simulink model "Differential_steer_kinematic"  (R2020b)
settings: Solver=FixedStepAuto  StartTime=0.0  StopTime=1000  FixedStep=.0001  MinStep=1E-5  RelTol=1e-3
values from neighbouring files (symbols this model uses):
  delay = 0.15    [Jackal_kinematic_model.m]
undefined symbols (not defined in the file or in its folder): path
libraries: fuzblock x2, robotalgslib x1, simulink x1
settings Model: Creator=12248  LastModifiedBy=mcichon2
settings SFSimCC: CustomCodeUndefinedFunction=UseInterfaceOnly

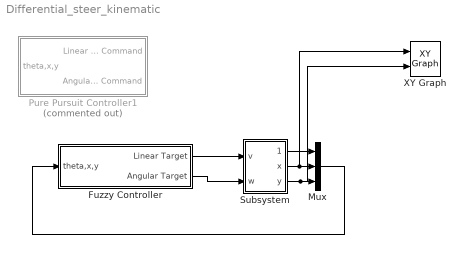
== system Differential_steer_kinematic ==
  Fuzzy Controller : Subsystem
  Mux : Mux  Inputs=3
  Pure Pursuit Controller1 : Subsystem  Commented=on
  Subsystem : Subsystem
  XY Graph : simulink/Sinks/XY Graph  xmin=-10  xmax=10  ymin=-10  ymax=10  st=-1
  wires:
  Mux/1 -> Fuzzy Controller/1(theta,x,y)
  Subsystem/1(theta) -> Mux/1
  Subsystem/2(x) -> XY Graph/1, Mux/2
  Subsystem/3(y) -> XY Graph/2, Mux/3
  Fuzzy Controller/1(Linear Target) -> Subsystem/1(v)
  Fuzzy Controller/2(" Angular Target") -> Subsystem/2(w)

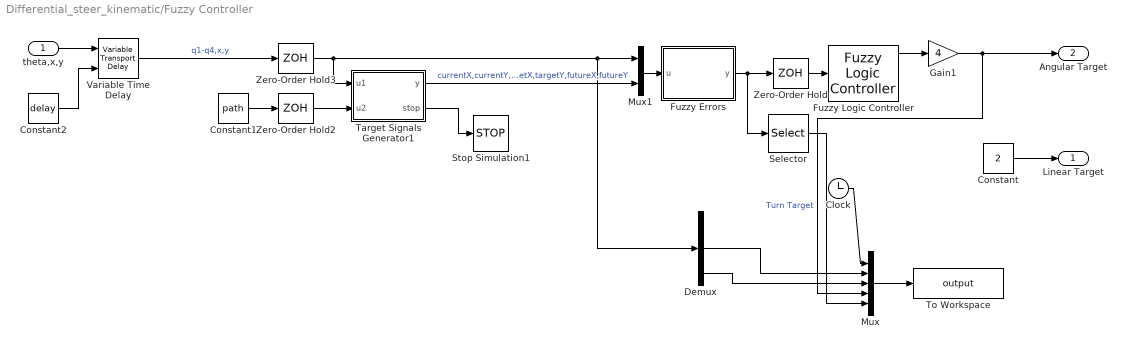
== system Differential_steer_kinematic/Fuzzy Controller ==
  theta,x,y : Inport
  Clock : Clock
  Constant : Constant  Value=2
  Constant1 : Constant  Value=path
  Constant2 : Constant  Value=delay
  Demux : Demux  Outputs=3
  Fuzzy Errors : MATLAB Function  TreatAsAtomicUnit=on
  Fuzzy Logic Controller : fuzblock/Fuzzy Logic  Controller  FIS='fuzzyControlDistNew.fis'  OutputSampleNumber=3000  DataType=double  FuzzifiedInputs=off  RuleFiringStrengths=on  RuleOutputs=off  AggregatedOutputs=on  SimulateUsing=Code generation  OutOfRangeInputValueMessage=warning  NoRuleFiredMessage=warning  EmptyOutputFuzzySetMessage=warning
  Gain1 : Gain  Gain=4
  Mux : Mux  Inputs=5
  Mux1 : Mux  Inputs=2
  Selector : Selector  InputPortWidth=5  IndexOptions=Index vector (dialog)  Indices=[1]  OutputSizes=1
  Stop Simulation1 : Stop
  Target Signals Generator1 : MATLAB Function  TreatAsAtomicUnit=on
  To Workspace : ToWorkspace  VariableName=output  SampleTime=-1
  Variable Time Delay : VariableTransportDelay  MaximumDelay=10
  Zero-Order Hold : ZeroOrderHold  SampleTime=.001
  Zero-Order Hold2 : ZeroOrderHold  SampleTime=.001
  Zero-Order Hold3 : ZeroOrderHold  SampleTime=.001
  Linear Target : Outport  VectorParamsAs1DForOutWhenUnconnected=off
  " Angular Target" : Outport  Port=2  VectorParamsAs1DForOutWhenUnconnected=off
  wires:
  Mux1/1 -> Fuzzy Errors/1(u)
  Variable Time Delay/1 -> Zero-Order Hold3/1  "q1-q4,x,y"
  Target Signals Generator1/1(y) -> Mux1/2  "currentX,currentY,targetX,targetY,futureX,futureY"
  Constant1/1 -> Zero-Order Hold2/1
  Zero-Order Hold2/1 -> Target Signals Generator1/2(u2)
  Target Signals Generator1/2(stop) -> Stop Simulation1/1
  Fuzzy Errors/1(y) -> Selector/1, Zero-Order Hold/1
  Zero-Order Hold/1 -> Fuzzy Logic Controller/1
  Fuzzy Logic Controller/1 -> Gain1/1
  Gain1/1 -> Mux/4, " Angular Target"/1  "Turn Target"
  theta,x,y/1 -> Variable Time Delay/1
  Constant/1 -> Linear Target/1
  Selector/1 -> Mux/5
  Mux/1 -> To Workspace/1
  Zero-Order Hold3/1 -> Target Signals Generator1/1(u1), Demux/1, Mux1/1
  Constant2/1 -> Variable Time Delay/2
  Clock/1 -> Mux/1
  Demux/2 -> Mux/2
  Demux/3 -> Mux/3

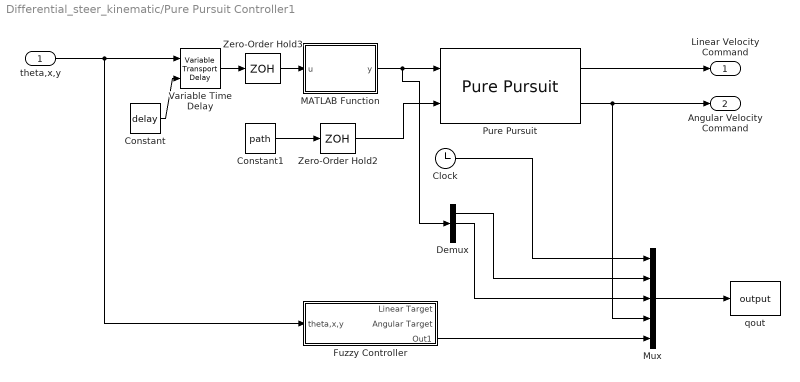
== system Differential_steer_kinematic/Pure Pursuit Controller1 ==
  theta,x,y : Inport
  Clock : Clock
  Constant : Constant  Value=delay
  Constant1 : Constant  Value=path
  Demux : Demux  Outputs=3
  Fuzzy Controller : Subsystem
  MATLAB Function : MATLAB Function  TreatAsAtomicUnit=on
  Mux : Mux  Inputs=5
  Pure Pursuit : robotalgslib/Pure Pursuit  DesiredLinearVelocity=speed  MaxAngularVelocity=4.0  LookaheadDistance=la_dist  TargetDirPort=off  SimulateUsing=Code generation
  Variable Time Delay : VariableTransportDelay  MaximumDelay=10
  Zero-Order Hold2 : ZeroOrderHold  SampleTime=.001
  Zero-Order Hold3 : ZeroOrderHold  SampleTime=.001
  qout : ToWorkspace  VariableName=output  SampleTime=-1
  Linear Velocity Command : Outport  VectorParamsAs1DForOutWhenUnconnected=off
  Angular Velocity Command : Outport  Port=2  VectorParamsAs1DForOutWhenUnconnected=off
  wires:
  Zero-Order Hold3/1 -> MATLAB Function/1(u)
  Constant1/1 -> Zero-Order Hold2/1
  MATLAB Function/1(y) -> Demux/1, Pure Pursuit/1
  Zero-Order Hold2/1 -> Pure Pursuit/2
  Pure Pursuit/2 -> Angular Velocity Command/1, Mux/4
  Variable Time Delay/1 -> Zero-Order Hold3/1
  Pure Pursuit/1 -> Linear Velocity Command/1
  Constant/1 -> Variable Time Delay/2
  Mux/1 -> qout/1
  Clock/1 -> Mux/1
  Fuzzy Controller/3(Out1) -> Mux/5
  theta,x,y/1 -> Fuzzy Controller/1(theta,x,y), Variable Time Delay/1
  Demux/1 -> Mux/2
  Demux/2 -> Mux/3

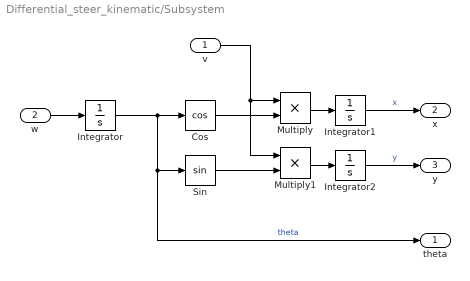
== system Differential_steer_kinematic/Subsystem ==
  v : Inport
  w : Inport  Port=2
  Cos : Trigonometry  Operator=cos
  Integrator : Integrator
  Integrator1 : Integrator
  Integrator2 : Integrator
  Multiply : Product
  Multiply1 : Product
  Sin : Trigonometry
  theta : Outport  VectorParamsAs1DForOutWhenUnconnected=off
  x : Outport  Port=2  VectorParamsAs1DForOutWhenUnconnected=off
  y : Outport  Port=3  VectorParamsAs1DForOutWhenUnconnected=off
  wires:
  Sin/1 -> Multiply1/2
  Multiply1/1 -> Integrator2/1
  Integrator/1 -> theta/1, Sin/1, Cos/1  "theta"
  Cos/1 -> Multiply/2
  Multiply/1 -> Integrator1/1
  Integrator1/1 -> x/1  "x"
  Integrator2/1 -> y/1  "y"
  v/1 -> Multiply1/1, Multiply/1
  w/1 -> Integrator/1

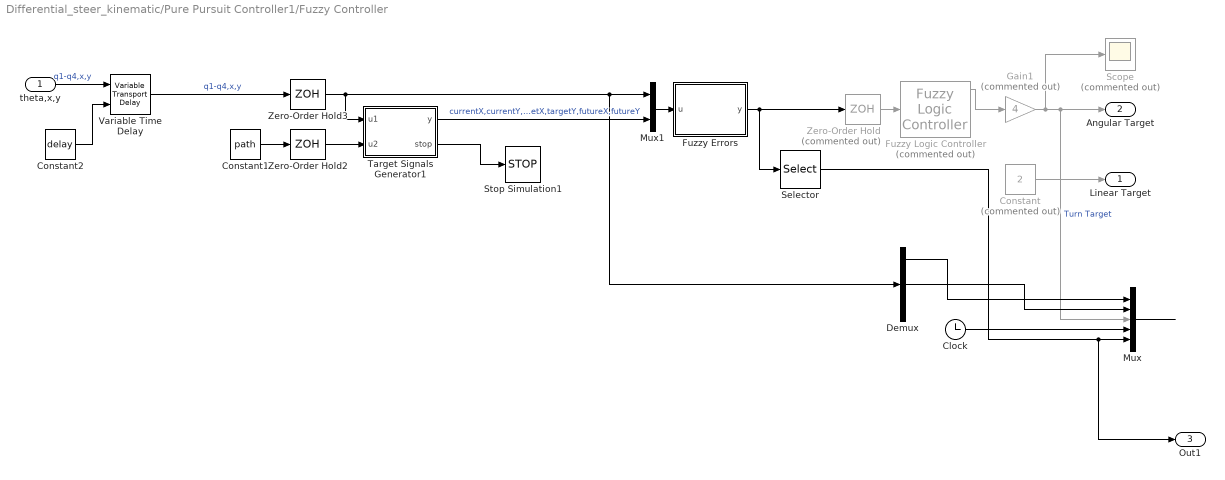
== system Differential_steer_kinematic/Pure Pursuit Controller1/Fuzzy Controller ==
  theta,x,y : Inport
  Clock : Clock
  Constant : Constant  Commented=on  Value=2
  Constant1 : Constant  Value=path
  Constant2 : Constant  Value=delay
  Demux : Demux  Outputs=3
  Fuzzy Errors : MATLAB Function  TreatAsAtomicUnit=on
  Fuzzy Logic Controller : fuzblock/Fuzzy Logic  Controller  Commented=on  FIS='fuzzyControlDistNew.fis'  OutputSampleNumber=3000  DataType=double  FuzzifiedInputs=off  RuleFiringStrengths=on  RuleOutputs=off  AggregatedOutputs=on  SimulateUsing=Code generation  OutOfRangeInputValueMessage=warning  NoRuleFiredMessage=warning  EmptyOutputFuzzySetMessage=warning
  Gain1 : Gain  Commented=on  Gain=4
  Mux : Mux  Inputs=5
  Mux1 : Mux  Inputs=2
  Scope : Scope  Commented=on
  Selector : Selector  InputPortWidth=5  IndexOptions=Index vector (dialog)  Indices=[1]  OutputSizes=1
  Stop Simulation1 : Stop
  Target Signals Generator1 : MATLAB Function  TreatAsAtomicUnit=on
  Variable Time Delay : VariableTransportDelay  MaximumDelay=10
  Zero-Order Hold : ZeroOrderHold  Commented=on  SampleTime=.001
  Zero-Order Hold2 : ZeroOrderHold  SampleTime=.001
  Zero-Order Hold3 : ZeroOrderHold  SampleTime=.001
  Linear Target : Outport  VectorParamsAs1DForOutWhenUnconnected=off
  " Angular Target" : Outport  Port=2  VectorParamsAs1DForOutWhenUnconnected=off
  Out1 : Outport  Port=3
  wires:
  Mux1/1 -> Fuzzy Errors/1(u)
  Variable Time Delay/1 -> Zero-Order Hold3/1  "q1-q4,x,y"
  Target Signals Generator1/1(y) -> Mux1/2  "currentX,currentY,targetX,targetY,futureX,futureY"
  Constant1/1 -> Zero-Order Hold2/1
  Zero-Order Hold2/1 -> Target Signals Generator1/2(u2)
  Target Signals Generator1/2(stop) -> Stop Simulation1/1
  Fuzzy Errors/1(y) -> Selector/1, Zero-Order Hold/1
  Zero-Order Hold/1 -> Fuzzy Logic Controller/1
  Fuzzy Logic Controller/1 -> Gain1/1
  Gain1/1 -> Mux/3, " Angular Target"/1, Scope/1  "Turn Target"
  Constant/1 -> Linear Target/1
  Clock/1 -> Mux/4
  Selector/1 -> Out1/1, Mux/5
  Mux/1 -> ?
  Zero-Order Hold3/1 -> Target Signals Generator1/1(u1), Demux/1, Mux1/1
  Demux/1 -> Mux/1
  Demux/2 -> Mux/2
  Constant2/1 -> Variable Time Delay/2
  theta,x,y/1 -> Variable Time Delay/1  "q1-q4,x,y"

== matlab function Differential_steer_kinematic/Pure Pursuit Controller1/MATLAB Function ==
  data: u input; y output
function y = fcn(u)
%jackal dyanamic model
pos=[u(2) u(3)]; % [x,y]
%q=[u(1) u(2) u(3) u(4)]; % orientation quaternion
%currentAngle=atan2(2*(q(1)*q(4)+q(2)*q(3)),1-2*(q(3)^2+q(4)^2));% Angle robot is currently facing
currentAngle=u(1);
y = [pos currentAngle];

== matlab function Differential_steer_kinematic/Fuzzy Controller/Target Signals Generator1 ==
  data: u1 input; y output; u2 input; stop output
function [y,stop] = fcn(u1,u2)

persistent pathcount;
persistent pathlength;
persistent path; %error in code, initially used path but this is already a matlab function
persistent pathPre;

if isempty(pathcount)
   pathcount=1;     
   pathPre=u2;
   [pathlength,~]=size(pathPre);  
   path=[pathPre; pathPre(pathlength,1)+100 pathPre(pathlength,2)+100]; %sim takes multiple iterations to stop after reaching final point, so this prevents it from breaking
end

pos=[u1(2) u1(3)]; % [x,y] 
currentPoint=path(pathcount,:);
target=path(pathcount+1,:);

A = [(currentPoint(2)-target(2)), target(1)-currentPoint(1); target(1)-currentPoint(1), target(2)-currentPoint(2)];
b = [ target(1)*currentPoint(2)-currentPoint(1)*target(2); pos(1)*(target(1)-currentPoint(1)) + pos(2)*(target(2)-currentPoint(2))];
proj = (A\b)'; %projected point on the line between  .
projLen=dot(proj-currentPoint,target-currentPoint)/norm(target-currentPoint)^2; %the distance along the projected line, where 0 is the start point and 1 is the end point

if ((projLen>1))
    pathcount=pathcount+1;
end

%check if at destination and terminate sim if there
pathflag=0;
if (pathcount==pathlength)
    
    pathflag=1;
end

if ((pathcount==(pathlength-1))||(pathcount==(pathlength)))
    a=path(pathcount,:);
    b=path(pathcount+1,:);
    post=path(pathcount+1,:);
else
    a=path(pathcount,:);
    b=path(pathcount+1,:);
    post=path(pathcount+2,:);
end

y = [a(1);a(2);b(1);b(2);post(1);post(2)];
stop=pathflag;

== matlab function Differential_steer_kinematic/Pure Pursuit Controller1/Fuzzy Controller/Fuzzy Errors ==
  settings: updateMethod=DISCRETE
  data: u input; y output
function y  = fcn(u)

%jackal dyanamic model
pos=[u(2) u(3)]; % [x,y]
%q=[u(1) u(2) u(3) u(4)]; % orientation quaternion
currentAngle=u(1);% Angle robot is currently facing

currentPoint=[u(4) u(5)];
target=[u(6) u(7)];
future=[u(8) u(9)];

A = [(currentPoint(2)-target(2)), target(1)-currentPoint(1); target(1)-currentPoint(1), target(2)-currentPoint(2)];
b = [ target(1)*currentPoint(2)-currentPoint(1)*target(2); pos(1)*(target(1)-currentPoint(1)) + pos(2)*(target(2)-currentPoint(2))];
proj = (A\b)'; %projected point on the line between  .

d = ( pos(1)-currentPoint(1) )*(target(2)-currentPoint(2)) - (pos(2)-currentPoint(2))*(target(1)-currentPoint(1));

if ( d >0)
    side = 1;
elseif ( d < 0)
    side = -1;
else
    side = 0;
end

distanceLine=norm(pos-proj)*side;
distanceTarget=sqrt((target(1)-pos(1))^2+(target(2)-pos(2))^2);

%wrap to +/-pi
if((currentAngle < -pi) || (pi < currentAngle))
    currentAngle = mod(currentAngle+pi, 2*pi)-pi;
end

farTarget=[.95*proj(1)+.05*target(1) .95*proj(2)+.05*target(2)];

th1 = atan2(farTarget(2)-pos(2), farTarget(1)-pos(1));
th2 = atan2(target(2)-currentPoint(2), target(1)-currentPoint(1));
th3 = atan2(future(2)-target(2), future(1)-target(1)); 

ThetaFar=th1-currentAngle;
ThetaNear=th2-currentAngle;
ThetaLookahead=th3-currentAngle;

%wrap to +/-pi
if((ThetaFar < -pi) || (pi < ThetaFar))
    ThetaFar = mod(ThetaFar+pi, 2*pi)-pi;
end

%wrap to +/-pi
if((ThetaNear < -pi) || (pi < ThetaNear))
    ThetaNear = mod(ThetaNear+pi, 2*pi)-pi;
end

%wrap to +/-pi
if((ThetaLookahead < -pi) || (pi < ThetaLookahead))
    ThetaLookahead = mod(ThetaLookahead+pi, 2*pi)-pi;
end

y = [distanceLine;ThetaFar;ThetaNear;ThetaLookahead;distanceTarget];

== matlab function Differential_steer_kinematic/Pure Pursuit Controller1/Fuzzy Controller/Target Signals Generator1 ==
  data: u1 input; y output; u2 input; stop output
function [y,stop] = fcn(u1,u2)

persistent pathcount;
persistent pathlength;
persistent path; %error in code, initially used path but this is already a matlab function
persistent pathPre;

if isempty(pathcount)
   pathcount=1;     
   pathPre=u2;
   [pathlength,~]=size(pathPre);  
   path=[pathPre; pathPre(pathlength,1)+100 pathPre(pathlength,2)+100]; %sim takes multiple iterations to stop after reaching final point, so this prevents it from breaking
end

pos=[u1(2) u1(3)]; % [x,y] 
currentPoint=path(pathcount,:);
target=path(pathcount+1,:);

A = [(currentPoint(2)-target(2)), target(1)-currentPoint(1); target(1)-currentPoint(1), target(2)-currentPoint(2)];
b = [ target(1)*currentPoint(2)-currentPoint(1)*target(2); pos(1)*(target(1)-currentPoint(1)) + pos(2)*(target(2)-currentPoint(2))];
proj = (A\b)'; %projected point on the line between  .
projLen=dot(proj-currentPoint,target-currentPoint)/norm(target-currentPoint)^2; %the distance along the projected line, where 0 is the start point and 1 is the end point

if ((projLen>1))
    pathcount=pathcount+1;
end

%check if at destination and terminate sim if there
pathflag=0;
if (pathcount==pathlength)
    
    pathflag=1;
end

if ((pathcount==(pathlength-1))||(pathcount==(pathlength)))
    a=path(pathcount,:);
    b=path(pathcount+1,:);
    post=path(pathcount+1,:);
else
    a=path(pathcount,:);
    b=path(pathcount+1,:);
    post=path(pathcount+2,:);
end

y = [a(1);a(2);b(1);b(2);post(1);post(2)];
stop=pathflag;

== matlab function Differential_steer_kinematic/Fuzzy Controller/Fuzzy Errors ==
  settings: updateMethod=DISCRETE
  data: u input; y output
function y  = fcn(u)

%jackal dyanamic model
pos=[u(2) u(3)]; % [x,y]
%q=[u(1) u(2) u(3) u(4)]; % orientation quaternion
%currentAngle=atan2(2*(q(1)*q(4)+q(2)*q(3)),1-2*(q(3)^2+q(4)^2));% Angle robot is currently facing
currentAngle=u(1);


currentPoint=[u(4) u(5)];
target=[u(6) u(7)];
future=[u(8) u(9)];

A = [(currentPoint(2)-target(2)), target(1)-currentPoint(1); target(1)-currentPoint(1), target(2)-currentPoint(2)];
b = [ target(1)*currentPoint(2)-currentPoint(1)*target(2); pos(1)*(target(1)-currentPoint(1)) + pos(2)*(target(2)-currentPoint(2))];
proj = (A\b)'; %projected point on the line between  .

d = ( pos(1)-currentPoint(1) )*(target(2)-currentPoint(2)) - (pos(2)-currentPoint(2))*(target(1)-currentPoint(1));

if ( d >0)
    side = 1;
elseif ( d < 0)
    side = -1;
else
    side = 0;
end

distanceLine=norm(pos-proj)*side;
distanceTarget=sqrt((target(1)-pos(1))^2+(target(2)-pos(2))^2);

%wrap to +/-pi
if((currentAngle < -pi) || (pi < currentAngle))
    currentAngle = mod(currentAngle+pi, 2*pi)-pi;
end

farTarget=[.95*proj(1)+.05*target(1) .95*proj(2)+.05*target(2)];

th1 = atan2(farTarget(2)-pos(2), farTarget(1)-pos(1));
th2 = atan2(target(2)-currentPoint(2), target(1)-currentPoint(1));
th3 = atan2(future(2)-target(2), future(1)-target(1)); 

ThetaFar=th1-currentAngle;
ThetaNear=th2-currentAngle;
ThetaLookahead=th3-currentAngle;

%wrap to +/-pi
if((ThetaFar < -pi) || (pi < ThetaFar))
    ThetaFar = mod(ThetaFar+pi, 2*pi)-pi;
end

%wrap to +/-pi
if((ThetaNear < -pi) || (pi < ThetaNear))
    ThetaNear = mod(ThetaNear+pi, 2*pi)-pi;
end

%wrap to +/-pi
if((ThetaLookahead < -pi) || (pi < ThetaLookahead))
    ThetaLookahead = mod(ThetaLookahead+pi, 2*pi)-pi;
end

y = [distanceLine;ThetaFar;ThetaNear;ThetaLookahead;distanceTarget];
